simulink model "TV_2017old"  (R2016a)
settings: Solver=FixedStepAuto  StartTime=0.0  StopTime=inf  FixedStep=0.001  RelTol=1e-3
PreLoadFcn:
  | TV_2017_parameters
values from neighbouring files (symbols this model uses):
  battery_voltage = single(530)    [HIL_parameters.m]    (also in HIL_parameters_2018.m; TV_2017_parameters.m; TV_2017_parameters_VD.m)
  car_params = Simulink_Car_params    [HIL_parameters.m]    (also in HIL_parameters_2018.m; TV_2017_parameters.m; TV_2017_parameters_VD.m)
  i_Diff = 16    [HIL_parameters.m]    (also in HIL_parameters_2018.m; TV_2017_parameters.m)
  Kp = 1    [HIL_parameters.m]    (also in HIL_parameters_2018.m; TV_2017_parameters.m; TV_2017_parameters_VD.m)
  motor_data = struct    [HIL_parameters.m]    (also in HIL_parameters_2018.m; TV_2017_parameters.m)
  powerLimitControl = Simulink_el    [HIL_parameters.m]    (also in HIL_parameters_2018.m; TV_2017_parameters.m; TV_2017_parameters_VD.m)
  settings = Simulink_Settings    [HIL_parameters.m]    (also in HIL_parameters_2018.m; TV_2017_parameters.m; TV_2017_parameters_VD.m)
  SpdC_BCC = 0    [HIL_parameters.m]    (also in HIL_parameters_2018.m; TV_2017_parameters.m; TV_2017_parameters_VD.m)
  Speed_Neg_sat = -21    [HIL_parameters.m]    (also in HIL_parameters_2018.m; TV_2017_parameters.m; TV_2017_parameters_VD.m)
  Speed_Pos_sat = 21    [HIL_parameters.m]    (also in HIL_parameters_2018.m; TV_2017_parameters.m; TV_2017_parameters_VD.m)
  SteeringAngleFL = [-23.80 -22.65 -21.50 -20.34 -19.18 -18.03 -16.86 -15.70 -14.53 -13.35 -12.18 -10.99 -9.80 -8.61 -7.40 -6.19 -4.97 -3.75 -2.51 -1.26 0 1.27 2.56 3.85 5.17 6.50 7.84 9.21 10.59 12.00 13.42 14.88 16.36 17.87 19.41 20.99 22.61 24.26 25.97 27.73 29.54]    [CarSetupAnalysis2018.m]    (also in HIL_parameters_2018.m; TV_2017_parameters.m; TV_2017_parameters_VD.m = [-24.129 -22.950 -21.772 -20.593 -19.413 -18.232 -17.050 -15)
  SteeringAngleFR = [-29.54 -27.73 -25.97 -24.26 -22.61 -20.99 -19.41 -17.87 -16.36 -14.88 -13.42 -12.00 -10.59 -9.21 -7.84 -6.50 -5.17 -3.85 -2.56 -1.27 0 1.26 2.51 3.75 4.97 6.19 7.40 8.61 9.80 10.99 12.18 13.35 14.53 15.70 16.86 18.03 19.18 20.34 21.50 22.65 23.80]    [CarSetupAnalysis2018.m]    (also in HIL_parameters_2018.m; TV_2017_parameters.m; TV_2017_parameters_VD.m = [-29.3050 -27.5340 -25.8140 -24.1410 -22.5110 -20.9180 -19.3)
  SteeringWhAngle = [-105 -99.75 -94.5 -89.25 -84 -78.75 -73.5 -68.25 -63 -57.75 -52.5 -47.25 -42 -36.75 -31.5 -26.25 -21.0 -15.75 -10.5 -5.25 0.0 5.25 10.50 15.75 21.00 26.25 31.50 36.75 42.00 47.25 52.50 57.75  63.00 68.25 73.50 78.75 84.00 89.25 94.50 99.75 105.00]    [TV_2017_parameters_VD.m]
  Tn_n = 0    [HIL_parameters.m]    (also in HIL_parameters_2018.m; TV_2017_parameters.m; TV_2017_parameters_VD.m)
  tractionControl = Simulink_tc    [HIL_parameters.m]    (also in HIL_parameters_2018.m; IterativeTractionControlTuning.m; TV_2017_parameters.m; TV_2017_parameters_VD.m)
  yawRateControl = Simulink_yawRate    [HIL_parameters.m]    (also in HIL_parameters_2018.m; TV_2017_parameters.m; TV_2017_parameters_VD.m)
undefined symbols (not defined in the file or in its folder): DiscIntNeverNeededParam, magnitude, speedEstimation, TC_Decr_Gas, TC_Derivative, TC_Incr_Gas, TC_On, TC_Relay_Off, TC_Relay_On
libraries: CarMaker4SL x274, simulink_extras x45, simulink x37, dspfdesign x2
(part 7 of 14)

== system TV_2017old/CarMaker/IPG Vehicle3/PowerTrain/Electric Powertrain/AMK RL ==
  Motor_speed_ref_in_RPM : Inport
  Whl_speed_rad_per_sec : Inport  Port=2
  "Torque_limit_pos " : Inport  Port=3
  Torque_limit_neg : Inport  Port=4
  Convert to RPM : Gain  Gain=60/(2*pi)
  Delay : Delay  DelayLength=3  InitialCondition=0
  Gain2 : Gain  Gain=-1
  Gear ratio : Gain  Gain=car_params.GR
  Gear ratio2 : Gain  Gain=car_params.GR
  Maximum torque output based on motor RPM : Lookup_n-D  NumberOfTableDimensions=1  BreakpointsForDimension1=motor_data.MaxTorqueBreakpoints  BreakpointsForDimension1Min=[0]  BreakpointsForDimension1Max=[20000]  Table=motor_data.MaxTorqueValues  ExtrapMethod=Clip  UseLastTableValue=on  InternalRulePriority=Speed  OutMin=[0]  OutMax=[21]  RndMeth=Simplest  InputSameDT=on
  Saturation : simulink/Discontinuities/Saturation Dynamic  OutMin=[]  OutMax=[]  OutDataTypeStr=Inherit: Same as second input  OutDataType=fixdt(1, 16)  OutScaling=2^-10  DoSatur=off
  Saturation Dynamic1 : simulink/Discontinuities/Saturation Dynamic  OutMin=[]  OutMax=[]  OutDataTypeStr=Inherit: Same as second input  OutDataType=fixdt(1, 16)  OutScaling=2^-10  DoSatur=off
  Speed PI 1 : simulink/Continuous/PID Controller  Controller=PI  TimeDomain=Discrete-time  SampleTime=-1  IntegratorMethod=Forward Euler  FilterMethod=Forward Euler  Form=Parallel  UseFilter=on  ControllerParametersSource=internal  P=Kp  I=Tn_n  D=0  N=100  InitialConditionSource=internal  InitialConditionForIntegrator=0  InitialConditionForFilter=0  ExternalReset=none  LimitOutput=on  UpperSaturationLimit=Speed_Pos_sat  LowerSaturationLimit=Speed_Neg_sat  LinearizeAsGain=off  AntiWindupMode=back-calculation  Kb=SpdC_BCC  TrackingMode=off  Kt=1  PParamMin=[]  PParamMax=[]  IParamMin=[]  IParamMax=[]  DParamMin=[]  DParamMax=[]  NParamMin=[]  NParamMax=[]  KbParamMin=[]  KbParamMax=[]  KtParamMin=[]  KtParamMax=[]  POutMin=[]  POutMax=[]  IOutMin=[]  IOutMax=[]  DOutMin=[]  DOutMax=[]  NOutMin=[]  NOutMax=[]  KbOutMin=[]  KbOutMax=[]  KtOutMin=[]  KtOutMax=[]  IntegratorOutMin=[]  IntegratorOutMax=[]  FilterOutMin=[]  FilterOutMax=[]  SumOutMin=[]  SumOutMax=[]  SumI1OutMin=[]  SumI1OutMax=[]  SumI2OutMin=[]  SumI2OutMax=[]  SumI3OutMin=[]  SumI3OutMax=[]  SumDOutMin=[]  SumDOutMax=[]  SaturationOutMin=[]  SaturationOutMax=[]  IntegratorContinuousStateAttributes=''  IntegratorStateMustResolveToSignalObject=off  IntegratorRTWStateStorageClass=Auto  FilterContinuousStateAttributes=''  FilterStateMustResolveToSignalObject=off  FilterRTWStateStorageClass=Auto  DifferentiatorICPrevScaledInput=0  DifferentiatorOutMin=[]  DifferentiatorOutMax=[]
  Sum : Sum  Inputs=|+-
  "Torque_Output " : Outport
  wires:
  Delay/1 -> "Torque_Output "/1
  Speed PI 1/1 -> Saturation/2
  Maximum torque output based on motor RPM/1 -> Saturation Dynamic1/1, Gain2/1
  Saturation Dynamic1/1 -> Gear ratio2/1
  Whl_speed_rad_per_sec/1 -> Gear ratio/1
  Gain2/1 -> Saturation Dynamic1/3
  Gear ratio2/1 -> Delay/1
  "Torque_limit_pos "/1 -> Saturation/1
  Torque_limit_neg/1 -> Saturation/3
  Motor_speed_ref_in_RPM/1 -> Sum/1
  Saturation/1 -> Saturation Dynamic1/2
  Sum/1 -> Speed PI 1/1
  Convert to RPM/1 -> Sum/2, Maximum torque output based on motor RPM/1
  Gear ratio/1 -> Convert to RPM/1

== system TV_2017old/CarMaker/IPG Vehicle3/PowerTrain/Electric Powertrain/AMK RR ==
  Motor_speed_ref_in_RPM : Inport
  Whl_speed_rad_per_sec : Inport  Port=2
  "Torque_limit_pos " : Inport  Port=3
  Torque_limit_neg : Inport  Port=4
  Convert to RPM : Gain  Gain=60/(2*pi)
  Delay : Delay  DelayLength=3  InitialCondition=0
  Gain2 : Gain  Gain=-1
  Gear ratio : Gain  Gain=car_params.GR
  Gear ratio2 : Gain  Gain=car_params.GR
  Maximum torque output based on motor RPM : Lookup_n-D  NumberOfTableDimensions=1  BreakpointsForDimension1=motor_data.MaxTorqueBreakpoints  BreakpointsForDimension1Min=[0]  BreakpointsForDimension1Max=[20000]  Table=motor_data.MaxTorqueValues  ExtrapMethod=Clip  UseLastTableValue=on  InternalRulePriority=Speed  OutMin=[0]  OutMax=[21]  RndMeth=Simplest  InputSameDT=on
  Saturation : simulink/Discontinuities/Saturation Dynamic  OutMin=[]  OutMax=[]  OutDataTypeStr=Inherit: Same as second input  OutDataType=fixdt(1, 16)  OutScaling=2^-10  DoSatur=off
  Saturation Dynamic1 : simulink/Discontinuities/Saturation Dynamic  OutMin=[]  OutMax=[]  OutDataTypeStr=Inherit: Same as second input  OutDataType=fixdt(1, 16)  OutScaling=2^-10  DoSatur=off
  Speed PI 1 : simulink/Continuous/PID Controller  Controller=PI  TimeDomain=Discrete-time  SampleTime=-1  IntegratorMethod=Forward Euler  FilterMethod=Forward Euler  Form=Parallel  UseFilter=on  ControllerParametersSource=internal  P=Kp  I=Tn_n  D=0  N=100  InitialConditionSource=internal  InitialConditionForIntegrator=0  InitialConditionForFilter=0  ExternalReset=none  LimitOutput=on  UpperSaturationLimit=Speed_Pos_sat  LowerSaturationLimit=Speed_Neg_sat  LinearizeAsGain=off  AntiWindupMode=back-calculation  Kb=SpdC_BCC  TrackingMode=off  Kt=1  PParamMin=[]  PParamMax=[]  IParamMin=[]  IParamMax=[]  DParamMin=[]  DParamMax=[]  NParamMin=[]  NParamMax=[]  KbParamMin=[]  KbParamMax=[]  KtParamMin=[]  KtParamMax=[]  POutMin=[]  POutMax=[]  IOutMin=[]  IOutMax=[]  DOutMin=[]  DOutMax=[]  NOutMin=[]  NOutMax=[]  KbOutMin=[]  KbOutMax=[]  KtOutMin=[]  KtOutMax=[]  IntegratorOutMin=[]  IntegratorOutMax=[]  FilterOutMin=[]  FilterOutMax=[]  SumOutMin=[]  SumOutMax=[]  SumI1OutMin=[]  SumI1OutMax=[]  SumI2OutMin=[]  SumI2OutMax=[]  SumI3OutMin=[]  SumI3OutMax=[]  SumDOutMin=[]  SumDOutMax=[]  SaturationOutMin=[]  SaturationOutMax=[]  IntegratorContinuousStateAttributes=''  IntegratorStateMustResolveToSignalObject=off  IntegratorRTWStateStorageClass=Auto  FilterContinuousStateAttributes=''  FilterStateMustResolveToSignalObject=off  FilterRTWStateStorageClass=Auto  DifferentiatorICPrevScaledInput=0  DifferentiatorOutMin=[]  DifferentiatorOutMax=[]
  Sum : Sum  Inputs=|+-
  "Torque_Output " : Outport
  wires:
  Gear ratio/1 -> Convert to RPM/1
  Convert to RPM/1 -> Maximum torque output based on motor RPM/1, Sum/2
  Sum/1 -> Speed PI 1/1
  Saturation/1 -> Saturation Dynamic1/2
  Motor_speed_ref_in_RPM/1 -> Sum/1
  Torque_limit_neg/1 -> Saturation/3
  "Torque_limit_pos "/1 -> Saturation/1
  Gear ratio2/1 -> Delay/1
  Gain2/1 -> Saturation Dynamic1/3
  Whl_speed_rad_per_sec/1 -> Gear ratio/1
  Saturation Dynamic1/1 -> Gear ratio2/1
  Maximum torque output based on motor RPM/1 -> Gain2/1, Saturation Dynamic1/1
  Speed PI 1/1 -> Saturation/2
  Delay/1 -> "Torque_Output "/1

== system TV_2017old/CarMaker/IPG Vehicle3/PowerTrain/Electric Powertrain/E-Gas // E-Motor ==
  VC.Gas : Inport
  Constant : Constant  Value=TC_On
  Constant1 : Constant  Value=TC_On
  E-Motor Mapping RL : Lookup2D  RowIndex=FSE_M85(1,2:end)  ColumnIndex=FSE_M85(2:end,1)  Table=FSE_M85(2:end,2:end)'  LookUpMeth=Interpolation-Use End Values
  E-Motor Mapping RR : Lookup2D  RowIndex=FSE_M85(1,2:end)  ColumnIndex=FSE_M85(2:end,1)  Table=FSE_M85(2:end,2:end)'  LookUpMeth=Interpolation-Use End Values
  Electronic Gas Pedal RL : Subsystem
  Electronic Gas Pedal RR : Subsystem
  Gain : Gain
  Gain1 : Gain
  Rotation RL : Subsystem
  Rotation RR : Subsystem
  Transfer Fcn : TransferFcn  Denominator=[0.015 1]
  Transfer Fcn1 : TransferFcn  Denominator=[0.015 1]
  Trq_RL : Outport
  Trq_RR : Outport  Port=2
  wires:
  Rotation RL/1(Engine_rot_RL) -> E-Motor Mapping RL/1
  Constant/1 -> Electronic Gas Pedal RL/1(TC_On)
  Electronic Gas Pedal RL/1(Motor_Gas_RL) -> E-Motor Mapping RL/2
  VC.Gas/1 -> Electronic Gas Pedal RL/2(VC.Gas), Electronic Gas Pedal RR/2(VC.Gas)
  Constant1/1 -> Electronic Gas Pedal RR/1(TC_On)
  E-Motor Mapping RL/1 -> Transfer Fcn/1
  Transfer Fcn/1 -> Gain/1
  Gain/1 -> Trq_RL/1
  Rotation RR/1(Engine_rot_RR) -> E-Motor Mapping RR/1
  Electronic Gas Pedal RR/1(Motor_Gas_RR) -> E-Motor Mapping RR/2
  Transfer Fcn1/1 -> Gain1/1
  E-Motor Mapping RR/1 -> Transfer Fcn1/1
  Gain1/1 -> Trq_RR/1

== system TV_2017old/CarMaker/IPG Vehicle3/PowerTrain/Electric Powertrain/Gas Pedal ==
  Clock : Clock
  Constant : Constant  Value=0
  Constant1 : Constant
  Fcn : Fcn  Expr=u==0
  Read CM Dict : CarMaker4SL/Read CM Dict  xname=Vhcl.Ignition  xsync=off
  Read CM Dict2 : CarMaker4SL/Read CM Dict  xname=VC.Gas  xsync=off
  Switch : Switch
  Switch1 : Switch
  Write CM Dict : CarMaker4SL/Write CM Dict  xname=Vhcl.Ignition  xsync=off
  VC.Gas : Outport
  wires:
  Read CM Dict2/1 -> Switch/1
  Switch/1 -> VC.Gas/1
  Constant/1 -> Switch/3
  Switch1/1 -> Switch/2, Write CM Dict/1
  Read CM Dict/1 -> Switch1/3
  Constant1/1 -> Switch1/1
  Fcn/1 -> Switch1/2
  Clock/1 -> Fcn/1

== system TV_2017old/CarMaker/IPG Vehicle3/CarAndTrailer/Forces/Tires/TireFL ==
  note: Insert your tire model here.
  Sync_In : Inport
  Load : Inport  Port=2
  vxtrans : Inport  Port=3
  vytrans : Inport  Port=4
  Rim_rotv : Inport  Port=5
  Rim_turnv : Inport  Port=6
  InclinAngle : Inport  Port=7
  muRoad : Inport  Port=8
  Ground{1..11} (11 alike) : Ground
  Terminator{,1..6,12} (8 alike) : Terminator
  Slp : Outport
  Alpha : Outport  Port=2
  TurnSlp : Outport  Port=3
  rBelt_eff : Outport  Port=4
  vBelt : Outport  Port=5
  LongFrc : Outport  Port=6
  SideFrc : Outport  Port=7
  LoadFrc : Outport  Port=8
  OverturnTrq : Outport  Port=9
  RollResist : Outport  Port=10
  AlignTrq : Outport  Port=11
  wires:
  Ground11/1 -> vBelt/1
  Ground10/1 -> rBelt_eff/1
  Ground9/1 -> TurnSlp/1
  Rim_turnv/1 -> Terminator6/1
  Sync_In/1 -> Terminator12/1
  Ground2/1 -> Alpha/1
  Ground3/1 -> LongFrc/1
  Ground4/1 -> SideFrc/1
  Ground5/1 -> OverturnTrq/1
  vxtrans/1 -> Terminator1/1
  vytrans/1 -> Terminator2/1
  Rim_rotv/1 -> Terminator3/1
  InclinAngle/1 -> Terminator4/1
  muRoad/1 -> Terminator5/1
  Load/1 -> Terminator/1
  Ground1/1 -> Slp/1
  Ground6/1 -> LoadFrc/1
  Ground7/1 -> RollResist/1
  Ground8/1 -> AlignTrq/1

== system TV_2017old/CarMaker/IPG Vehicle3/CarAndTrailer/Forces/Tires/TireFR ==
  note: Insert your tire model here.
  Sync_In : Inport
  Load : Inport  Port=2
  vxtrans : Inport  Port=3
  vytrans : Inport  Port=4
  Rim_rotv : Inport  Port=5
  Rim_turnv : Inport  Port=6
  InclinAngle : Inport  Port=7
  muRoad : Inport  Port=8
  Ground{1..11} (11 alike) : Ground
  Terminator{,1..6,12} (8 alike) : Terminator
  Slp : Outport
  Alpha : Outport  Port=2
  TurnSlp : Outport  Port=3
  rBelt_eff : Outport  Port=4
  vBelt : Outport  Port=5
  LongFrc : Outport  Port=6
  SideFrc : Outport  Port=7
  LoadFrc : Outport  Port=8
  OverturnTrq : Outport  Port=9
  RollResist : Outport  Port=10
  AlignTrq : Outport  Port=11
  wires:
  Ground11/1 -> vBelt/1
  Ground10/1 -> rBelt_eff/1
  Ground9/1 -> TurnSlp/1
  Rim_turnv/1 -> Terminator6/1
  Sync_In/1 -> Terminator12/1
  Ground2/1 -> Alpha/1
  Ground3/1 -> LongFrc/1
  Ground4/1 -> SideFrc/1
  Ground5/1 -> OverturnTrq/1
  vxtrans/1 -> Terminator1/1
  vytrans/1 -> Terminator2/1
  Rim_rotv/1 -> Terminator3/1
  InclinAngle/1 -> Terminator4/1
  muRoad/1 -> Terminator5/1
  Load/1 -> Terminator/1
  Ground1/1 -> Slp/1
  Ground6/1 -> LoadFrc/1
  Ground7/1 -> RollResist/1
  Ground8/1 -> AlignTrq/1

== system TV_2017old/CarMaker/IPG Vehicle3/CarAndTrailer/Forces/Tires/TireRL ==
  note: Insert your tire model here.
  Sync_In : Inport
  Load : Inport  Port=2
  vxtrans : Inport  Port=3
  vytrans : Inport  Port=4
  Rim_rotv : Inport  Port=5
  Rim_turnv : Inport  Port=6
  InclinAngle : Inport  Port=7
  muRoad : Inport  Port=8
  Ground{1..11} (11 alike) : Ground
  Terminator{,1..6,12} (8 alike) : Terminator
  Slp : Outport
  Alpha : Outport  Port=2
  TurnSlp : Outport  Port=3
  rBelt_eff : Outport  Port=4
  vBelt : Outport  Port=5
  LongFrc : Outport  Port=6
  SideFrc : Outport  Port=7
  LoadFrc : Outport  Port=8
  OverturnTrq : Outport  Port=9
  RollResist : Outport  Port=10
  AlignTrq : Outport  Port=11
  wires:
  Ground11/1 -> vBelt/1
  Ground10/1 -> rBelt_eff/1
  Ground9/1 -> TurnSlp/1
  Rim_turnv/1 -> Terminator6/1
  Sync_In/1 -> Terminator12/1
  Ground2/1 -> Alpha/1
  Ground3/1 -> LongFrc/1
  Ground4/1 -> SideFrc/1
  Ground5/1 -> OverturnTrq/1
  vxtrans/1 -> Terminator1/1
  vytrans/1 -> Terminator2/1
  Rim_rotv/1 -> Terminator3/1
  InclinAngle/1 -> Terminator4/1
  muRoad/1 -> Terminator5/1
  Load/1 -> Terminator/1
  Ground1/1 -> Slp/1
  Ground6/1 -> LoadFrc/1
  Ground7/1 -> RollResist/1
  Ground8/1 -> AlignTrq/1

== system TV_2017old/CarMaker/IPG Vehicle3/CarAndTrailer/Forces/Tires/TireRR ==
  note: Insert your tire model here.
  Sync_In : Inport
  Load : Inport  Port=2
  vxtrans : Inport  Port=3
  vytrans : Inport  Port=4
  Rim_rotv : Inport  Port=5
  Rim_turnv : Inport  Port=6
  InclinAngle : Inport  Port=7
  muRoad : Inport  Port=8
  Ground{1..11} (11 alike) : Ground
  Terminator{,1..6,12} (8 alike) : Terminator
  Slp : Outport
  Alpha : Outport  Port=2
  TurnSlp : Outport  Port=3
  rBelt_eff : Outport  Port=4
  vBelt : Outport  Port=5
  LongFrc : Outport  Port=6
  SideFrc : Outport  Port=7
  LoadFrc : Outport  Port=8
  OverturnTrq : Outport  Port=9
  RollResist : Outport  Port=10
  AlignTrq : Outport  Port=11
  wires:
  Ground11/1 -> vBelt/1
  Ground10/1 -> rBelt_eff/1
  Ground9/1 -> TurnSlp/1
  Rim_turnv/1 -> Terminator6/1
  Sync_In/1 -> Terminator12/1
  Ground2/1 -> Alpha/1
  Ground3/1 -> LongFrc/1
  Ground4/1 -> SideFrc/1
  Ground5/1 -> OverturnTrq/1
  vxtrans/1 -> Terminator1/1
  vytrans/1 -> Terminator2/1
  Rim_rotv/1 -> Terminator3/1
  InclinAngle/1 -> Terminator4/1
  muRoad/1 -> Terminator5/1
  Load/1 -> Terminator/1
  Ground1/1 -> Slp/1
  Ground6/1 -> LoadFrc/1
  Ground7/1 -> RollResist/1
  Ground8/1 -> AlignTrq/1

== system TV_2017old/CarMaker/IPG Vehicle3/PowerTrain/Electric Powertrain/E-Gas // E-Motor/Electronic Gas Pedal RL ==
  TC_On : Inport
  VC.Gas : Inport  Port=2
  Define CM Dict : CarMaker4SL/Define CM Dict  xname=E_Gas_RL  xmono=off  xtype=Double4  xdvaplace=None  xnstates=0  xfirststate=0  xinitial=0
  Read CM Dict1 : CarMaker4SL/Read CM Dict  xname=E_Gas_RL  xsync=off
  Read CM Dict2 : CarMaker4SL/Read CM Dict  xname=Car.LongSlipRL  xsync=off
  Subsystem1 : Subsystem
  Switch : Switch
  Write CM Dict : CarMaker4SL/Write CM Dict  xname=E_Gas_RL  xsync=off
  Motor_Gas_RL : Outport
  wires:
  VC.Gas/1 -> Switch/3, Subsystem1/1(VC.Gas)
  Switch/1 -> Motor_Gas_RL/1
  TC_On/1 -> Switch/2
  Subsystem1/1(E_Gas) -> Write CM Dict/1, Switch/1
  Read CM Dict1/1 -> Subsystem1/2(E_Gas.)
  Read CM Dict2/1 -> Subsystem1/3(Car.LongSlip)

== system TV_2017old/CarMaker/IPG Vehicle3/PowerTrain/Electric Powertrain/E-Gas // E-Motor/Electronic Gas Pedal RR ==
  TC_On : Inport
  VC.Gas : Inport  Port=2
  Define CM Dict : CarMaker4SL/Define CM Dict  xname=E_Gas_RR  xmono=off  xtype=Double4  xdvaplace=None  xnstates=0  xfirststate=0  xinitial=0
  Read CM Dict1 : CarMaker4SL/Read CM Dict  xname=E_Gas_RR  xsync=off
  Read CM Dict2 : CarMaker4SL/Read CM Dict  xname=Car.LongSlipRR  xsync=off
  Subsystem1 : Subsystem
  Switch : Switch
  Write CM Dict : CarMaker4SL/Write CM Dict  xname=E_Gas_RR  xsync=off
  Motor_Gas_RR : Outport
  wires:
  TC_On/1 -> Switch/2
  Switch/1 -> Motor_Gas_RR/1
  VC.Gas/1 -> Switch/3, Subsystem1/1(VC.Gas)
  Subsystem1/1(E_Gas) -> Write CM Dict/1, Switch/1
  Read CM Dict2/1 -> Subsystem1/3(Car.LongSlip)
  Read CM Dict1/1 -> Subsystem1/2(E_Gas.)

== system TV_2017old/CarMaker/IPG Vehicle3/PowerTrain/Electric Powertrain/E-Gas // E-Motor/Rotation RL ==
  Gain : Gain  Gain=i_Diff
  Gain1 : Gain  Gain=60/(2*pi)
  Read CM Dict : CarMaker4SL/Read CM Dict  xname=Car.WheelSpd_RL  xsync=off
  Engine_rot_RL : Outport
  wires:
  Read CM Dict/1 -> Gain/1
  Gain/1 -> Gain1/1
  Gain1/1 -> Engine_rot_RL/1

== system TV_2017old/CarMaker/IPG Vehicle3/PowerTrain/Electric Powertrain/E-Gas // E-Motor/Rotation RR ==
  Gain : Gain  Gain=i_Diff
  Gain1 : Gain  Gain=60/(2*pi)
  Read CM Dict : CarMaker4SL/Read CM Dict  xname=Car.WheelSpd_RR  xsync=off
  Engine_rot_RR : Outport
  wires:
  Gain1/1 -> Engine_rot_RR/1
  Gain/1 -> Gain1/1
  Read CM Dict/1 -> Gain/1

== system TV_2017old/CarMaker/IPG Vehicle3/PowerTrain/Electric Powertrain/E-Gas // E-Motor/Electronic Gas Pedal RL/Subsystem1 ==
  VC.Gas : Inport
  E_Gas. : Inport  Port=2
  Car.LongSlip : Inport  Port=3
  Add : Sum
  Compare To Constant : simulink/Logic and Bit Operations/Compare To Constant  relop=>  const=TC_Derivative  OutDataTypeStr=uint8  ZeroCross=off
  Derivative : Derivative
  Fcn : Fcn  Expr=u >0.05
  Fcn1 : Fcn  Expr=u+TC_Incr_Gas
  Fcn2 : Fcn  Expr=u-TC_Decr_Gas
  Multiport Switch : MultiPortSwitch  DataPortOrder=Zero-based contiguous  zeroidx=on
  Relational Operator : RelationalOperator  Operator=<=
  Relay : Relay  OnSwitchValue=TC_Relay_On  OffSwitchValue=TC_Relay_Off
  S-R Flip-Flop : simulink_extras/Flip Flops/S-R Flip-Flop  initial_condition=0
  Saturation : Saturate  UpperLimit=1  LowerLimit=0
  Saturation1 : Saturate  UpperLimit=1  LowerLimit=0
  Switch : Switch  Criteria=u2 > Threshold
  Terminator : Terminator
  E_Gas : Outport
  wires:
  Car.LongSlip/1 -> Relay/1, Derivative/1, Fcn/1
  Relay/1 -> Add/1
  Derivative/1 -> Compare To Constant/1
  Compare To Constant/1 -> Add/2
  Add/1 -> Multiport Switch/1
  Multiport Switch/1 -> E_Gas/1
  VC.Gas/1 -> Relational Operator/1, [A]
  E_Gas./1 -> Relational Operator/2, Fcn1/1, Fcn2/1, Multiport Switch/3
  S-R Flip-Flop/2 -> Terminator/1
  S-R Flip-Flop/1 -> Switch/2
  Switch/1 -> Multiport Switch/2
  Fcn/1 -> S-R Flip-Flop/1
  Relational Operator/1 -> S-R Flip-Flop/2
  Fcn1/1 -> Saturation1/1
  Saturation1/1 -> Switch/1
  Fcn2/1 -> Saturation/1
  Saturation/1 -> Multiport Switch/4
  [A] -> Switch/3

== system TV_2017old/CarMaker/IPG Vehicle3/PowerTrain/Electric Powertrain/E-Gas // E-Motor/Electronic Gas Pedal RR/Subsystem1 ==
  VC.Gas : Inport
  E_Gas. : Inport  Port=2
  Car.LongSlip : Inport  Port=3
  Add : Sum
  Compare To Constant : simulink/Logic and Bit Operations/Compare To Constant  relop=>  const=TC_Derivative  OutDataTypeStr=uint8  ZeroCross=off
  Derivative : Derivative
  Fcn : Fcn  Expr=u >0.05
  Fcn1 : Fcn  Expr=u+TC_Incr_Gas
  Fcn2 : Fcn  Expr=u-TC_Decr_Gas
  Multiport Switch : MultiPortSwitch  DataPortOrder=Zero-based contiguous  zeroidx=on
  Relational Operator : RelationalOperator  Operator=<=  InputSameDT=on
  Relay : Relay  OnSwitchValue=TC_Relay_On  OffSwitchValue=TC_Relay_Off
  S-R Flip-Flop : simulink_extras/Flip Flops/S-R Flip-Flop  initial_condition=0
  Saturation : Saturate  UpperLimit=1  LowerLimit=0
  Saturation1 : Saturate  UpperLimit=1  LowerLimit=0
  Switch : Switch  Criteria=u2 > Threshold
  Terminator : Terminator
  E_Gas : Outport
  wires:
  Car.LongSlip/1 -> Relay/1, Derivative/1, Fcn/1
  Relay/1 -> Add/1
  Derivative/1 -> Compare To Constant/1
  Compare To Constant/1 -> Add/2
  Add/1 -> Multiport Switch/1
  Multiport Switch/1 -> E_Gas/1
  VC.Gas/1 -> Relational Operator/1, [A]
  E_Gas./1 -> Relational Operator/2, Fcn1/1, Fcn2/1, Multiport Switch/3
  S-R Flip-Flop/2 -> Terminator/1
  S-R Flip-Flop/1 -> Switch/2
  Switch/1 -> Multiport Switch/2
  Fcn/1 -> S-R Flip-Flop/1
  Relational Operator/1 -> S-R Flip-Flop/2
  Fcn1/1 -> Saturation1/1
  Saturation1/1 -> Switch/1
  Fcn2/1 -> Saturation/1
  Saturation/1 -> Multiport Switch/4
  [A] -> Switch/3

== matlab function TV_2017old/CarMaker/Control_System /Power Limit Torque Reduction Controller /Old powerlimiting /extractPower1 ==
  data: states input; power output; powerLimitControl parameter
function power = extractPower(states,powerLimitControl)
%#codegen


if (powerLimitControl.enable == uint32(1))
    power = states.power;
else
    power = single(0);
end

end

== matlab function TV_2017old/CarMaker/Control_System /Yaw Rate Controller /yawRateReference ==
  data: r_der_error output; r_error output; vx output; states input Bus: States; prev_r_error input; r_ref output; yawRateControl parameter; car_params parameter; r_lim output; ay_max output; settings parameter
function [r_der_error,r_error, vx, r_ref,r_lim,ay_max]...
          = yawrate_reference(states,prev_r_error, yawRateControl, car_params,settings)

%#codegen
updatefactor = single(1);
r_lim = single(0);
ay_max = single(0);
delta = states.wheel_angle;
delta_der = states.wheel_speed;
% If Ku is negative there will be a problem if the denominator approaches
% zero at high speeds
r_ref = (states.V_x/(yawRateControl.r_ref_tuning_param + yawRateControl.Ku*states.V_x^2))*tan(delta); %  tan

%r_ref = (states.V_x/(yawRateControl.r_ref_tuning_param*(1 + yawRateControl.Ku*states.V_x^2)))* delta;

%Fzi = [states.Fz_FL states.Fz_FR states.Fz_RL states.Fz_RR];
if yawRateControl.enable_r_ref_limit == 1
    r_lim = settings.mu*yawRateControl.mu_scaling_r_ref_limit*9.81/states.V_x;
    if abs(r_ref) > abs(r_lim)
        r_ref = r_lim*sign(r_ref);
    end
end

r = states.r;
r_error = prev_r_error*(1-updatefactor) + updatefactor*(r_ref-r);
r_ref_der = (states.ax*delta + states.V_x*delta_der)/yawRateControl.r_ref_tuning_param;
r_der_error = r_ref_der*yawRateControl.ref_weight - states.r_der*yawRateControl.meas_weight;

vx = states.V_x;
end

== matlab function TV_2017old/CarMaker/Control_System /Slip Rate Control /Traction Controllers/MATLAB Function1 ==
  data: states input Bus: States; SR_FL output; SR_FR output; SR_RL output; SR_RR output; T_req input; tractionControl parameter; Kp output; Ki output; settings parameter; T_tv input Bus: Ti_lim
function [SR_FL, SR_FR, SR_RL, SR_RR, Kp, Ki] = slipRatioAndGains(states, T_req, tractionControl, settings, T_tv)
%#codegen


SR_FL = states.SR_FL;
SR_FR = states.SR_FR;
SR_RL = states.SR_RL;
SR_RR = states.SR_RR;



if (states.V_x >= 0) 
    vx_kmh = states.V_x*3.6;
else
    vx_kmh = single(0);
end

    

a_kp = single((tractionControl.Kp_end - tractionControl.Kp_start) / tractionControl.lookup_speed_end_kmh);
a_ki = single((tractionControl.Ki_end - tractionControl.Ki_start) / tractionControl.lookup_speed_end_kmh);



if ( ( (T_req + 0.0001) > 0) && (vx_kmh < tractionControl.full_gain_limit_kmh) )   
    Kp = min( (a_kp*max(0,vx_kmh) + tractionControl.Kp_start), tractionControl.Kp_end)  * abs(T_req)/(settings.max_motor_torque*4);
    Ki = min( (a_ki*max(0,vx_kmh) + tractionControl.Ki_start), tractionControl.Ki_end)  * abs(T_req)/(settings.max_motor_torque*4);
else
    Kp = min( (a_kp*max(0,vx_kmh) + tractionControl.Kp_start), tractionControl.Kp_end);
    Ki = min( (a_ki*max(0,vx_kmh) + tractionControl.Ki_start), tractionControl.Ki_end);
end

end






% This one solves starting from 0 kmh with the driver controlling the
% throttle. This statement reduces the gains according to the requested
% torque, to avoid oscillating torque output


% if ( ( (T_req + 0.0001) > 0) && (vx_kmh < tractionControl.full_gain_limit_kmh) )   
%     Kp_driving = min( (a_kp*max(0,vx_kmh) + tractionControl.Kp_start), tractionControl.Kp_end)  * abs(T_req)/(settings.max_motor_torque*4);
%     Ki_driving = min( (a_ki*max(0,vx_kmh) + tractionControl.Ki_start), tractionControl.Ki_end)  * abs(T_req)/(settings.max_motor_torque*4);
%     Kp_FL = Kp_driving;
%     Kp_FR = Kp_driving;
%     Kp_RL = Kp_driving;
%     Kp_RR = Kp_driving;
%     
%     Ki_FL = Ki_driving;
%     Ki_FR = Ki_driving;
%     Ki_RL = Ki_driving;
%     Ki_RR = Ki_driving;
%     %Kp = min( (a_kp*max(0,vx_kmh) + tractionControl.Kp_start), tractionControl.Kp_end)  * abs(T_req)/(settings.max_motor_torque*4);
%     %Ki = min( (a_ki*max(0,vx_kmh) + tractionControl.Ki_start), tractionControl.Ki_end)  * abs(T_req)/(settings.max_motor_torque*4);
% 
% % T_req positive and speed over full gain limit
% elseif ( ( (T_req + 0.0001) > 0) && (vx_kmh > tractionControl.full_gain_limit_kmh))
%     Kp_driving = min( (a_kp*max(0,vx_kmh) + tractionControl.Kp_start), tractionControl.Kp_end);
%     Ki_driving = min( (a_ki*max(0,vx_kmh) + tractionControl.Ki_start), tractionControl.Ki_end);
%     Kp_FL = Kp_driving;
%     Kp_FR = Kp_driving;
%     Kp_RL = Kp_driving;
%     Kp_RR = Kp_driving;
%     
%     Ki_FL = Ki_driving;
%     Ki_FR = Ki_driving;
%     Ki_RL = Ki_driving;
%     Ki_RR = Ki_driving;    
% else   
%     Kp_FL = min( (a_kp*max(0,vx_kmh) + tractionControl.Kp_start), tractionControl.Kp_end);
%     Kp_FR = min( (a_kp*max(0,vx_kmh) + tractionControl.Kp_start), tractionControl.Kp_end);
%     Kp_RL = min( (a_kp*max(0,vx_kmh) + tractionControl.Kp_start), tractionControl.Kp_end);
%     Kp_RR = min( (a_kp*max(0,vx_kmh) + tractionControl.Kp_start), tractionControl.Kp_end);
%     
%     Ki_FL = min( (a_ki*max(0,vx_kmh) + tractionControl.Ki_start), tractionControl.Ki_end);
%     Ki_FR = min( (a_ki*max(0,vx_kmh) + tractionControl.Ki_start), tractionControl.Ki_end);
%     Ki_RL = min( (a_ki*max(0,vx_kmh) + tractionControl.Ki_start), tractionControl.Ki_end);
%     Ki_RR = min( (a_ki*max(0,vx_kmh) + tractionControl.Ki_start), tractionControl.Ki_end);
%     
%     %Kp = tractionControl.Kp_braking;
%     %Ki = tractionControl.Ki_braking;
% end
% 
% if ( (T_tv.FL < 0) || (T_tv.FR < 0) || (T_tv.RL < 0) || (T_tv.RR < 0) )
%     Kp = tractionControl.Kp_braking;
%     Ki = tractionControl.Ki_braking;
% end

== matlab function TV_2017old/CarMaker/Control_System /MATLAB Function3 ==
  data: Ti input Bus: Ti_lim; states input; Ti_pos output Bus: Ti_pos; Ti_neg output Bus: Ti_neg; wi_setpoints output Bus: wi_set; settings parameter; car_params parameter; overTorque output
function [Ti_pos, Ti_neg, wi_setpoints, overTorque] = setPointCalculation(Ti,states,settings,car_params)
%#codegen

%Conversion factor to calculate RPM limits based on speed limits
%v_to_motor_RPM = single(60*car_params.GR/(2*pi*car_params.r_eff));
overTorque = int8(0);
r = car_params.r_eff;
GR = car_params.GR;
scale_factor = 5;
not_in_use = settings.RPM_scaling;
max_rpm = settings.max_RPM;
KERS_RPM_setpoint = settings.KERS_motor_RPM_setpoint;
%scaled_RPM_lim_pos = states.V_x* (60/2*pi*r)*scale_factor;
v_x = states.V_x;
if v_x>5;
    scaled_RPM_lim_pos =  min([max_rpm ,GR*v_x* (60/2*pi*r)*scale_factor]);
else
   scaled_RPM_lim_pos = single( min([max_rpm ,GR*5* (60/2*pi*r)*scale_factor]));
end


if max([Ti.FL Ti.FR Ti.RL Ti.RR]) > (21+0.0001)
    %this is bad
    overTorque = int8(1);
end



 %***************** FL *********** 

if  (Ti.FL <= 0)  
    Ti_pos.FL = int16(0);
    Ti_neg.FL = int16(max(-settings.max_motor_brake_torque/car_params.Mn, Ti.FL/car_params.Mn));
    wi_setpoints.FL = int16(KERS_RPM_setpoint);

elseif Ti.FL > 0
    Ti_pos.FL = int16(min(21/car_params.Mn , Ti.FL/car_params.Mn));
    Ti_neg.FL = int16(0);
    wi_setpoints.FL = int16(max_rpm);  
else
    Ti_pos.FL = int16(0);
    Ti_neg.FL = int16(0);
    wi_setpoints.FL = int16(1); 
end

%***************** FR ************

if  (Ti.FR <= 0)
    Ti_pos.FR = int16(0);
    Ti_neg.FR = int16(max(-settings.max_motor_brake_torque/car_params.Mn, Ti.FR/car_params.Mn));
    wi_setpoints.FR = int16(KERS_RPM_setpoint);

elseif Ti.FR > 0        
    Ti_pos.FR = int16( min(21/car_params.Mn , Ti.FR/car_params.Mn));
    Ti_neg.FR = int16(0);
    wi_setpoints.FR = int16(max_rpm);  
else
    Ti_pos.FR = int16(0);
    Ti_neg.FR = int16(0);
    wi_setpoints.FR = int16(1); 
end
%***************** RL ************
if  (Ti.RL <= 0)
    Ti_pos.RL = int16(0);
    Ti_neg.RL = int16(max(-settings.max_motor_brake_torque/car_params.Mn, Ti.RL/car_params.Mn));
    wi_setpoints.RL = int16(KERS_RPM_setpoint);

elseif Ti.RL > 0
    Ti_pos.RL = int16(min(21/car_params.Mn , Ti.RL/car_params.Mn));
    Ti_neg.RL = int16(0);
    wi_setpoints.RL = int16(max_rpm);  
else
    Ti_pos.RL = int16(0);
    Ti_neg.RL = int16(0);
    wi_setpoints.RL = int16(1); 
end

%***************** RR ************
if (Ti.RR <= 0)
    Ti_pos.RR = int16(0);
    Ti_neg.RR = int16(max(-settings.max_motor_brake_torque/car_params.Mn, Ti.RR/car_params.Mn));
    wi_setpoints.RR = int16(KERS_RPM_setpoint);

elseif Ti.RR > 0
    Ti_pos.RR = int16(min(21/car_params.Mn , Ti.RR/car_params.Mn));
    Ti_neg.RR = int16(0);
    wi_setpoints.RR = int16(max_rpm);  
else
    Ti_pos.RR = int16(0);
    Ti_neg.RR = int16(0);
    wi_setpoints.RR = int16(1); 
end
end



% _________________________________________________________________________________________  
% 
% %***************** FL ************
% if dynamic_rpm ==1
%     if  (Ti.FL <= 0)  
%         Ti_pos.FL = int16(0);
%         Ti_neg.FL = int16(max(-settings.max_motor_brake_torque/car_params.Mn, Ti.FL/car_params.Mn));
%         wi_setpoints.FL = int16(KERS_RPM_setpoint);
% 
%     elseif Ti.FL > 0 
%         Ti_pos.FL = int16( Ti.FL/car_params.Mn);
%         Ti_neg.FL = int16(0);
%         wi_setpoints.FL = int16(scaled_RPM_lim_pos);  
%     else
%         Ti_pos.FL = int16(0);
%         Ti_neg.FL = int16(0);
%         wi_setpoints.FL = int16(2); 
%     end
% 
%     %***************** FR ************
% 
%     if  (Ti.FR <= 0)
%         Ti_pos.FR = int16(0);
%         Ti_neg.FR = int16(max(-settings.max_motor_brake_torque/car_params.Mn, Ti.FR/car_params.Mn));
%         wi_setpoints.FR = int16(KERS_RPM_setpoint);
% 
%     elseif Ti.FR > 0
%         Ti_pos.FR = int16( Ti.FR/car_params.Mn);
%         Ti_neg.FR = int16(0);
%         wi_setpoints.FR = int16(scaled_RPM_lim_pos);  
%     else
%         Ti_pos.FR = int16(0);
%         Ti_neg.FR = int16(0);
%         wi_setpoints.FR = int16(2); 
%     end
%     %***************** RL ************
%     if  (Ti.RL <= 0)
%         Ti_pos.RL = int16(0);
%         Ti_neg.RL = int16(max(-settings.max_motor_brake_torque/car_params.Mn, Ti.RL/car_params.Mn));
%         wi_setpoints.RL = int16(KERS_RPM_setpoint);
% 
%     elseif Ti.RL > 0
%         Ti_pos.RL = int16( Ti.RL/car_params.Mn);
%         Ti_neg.RL = int16(0);
%         wi_setpoints.RL = int16(scaled_RPM_lim_pos);  
%     else
%         Ti_pos.RL = int16(0);
%         Ti_neg.RL = int16(0);
%         wi_setpoints.RL = int16(2); 
%     end
% 
%     %***************** RR ************
%     if (Ti.RR <= 0)
%         Ti_pos.RR = int16(0);
%         Ti_neg.RR = int16(max(-settings.max_motor_brake_torque/car_params.Mn, Ti.RR/car_params.Mn));
%         wi_setpoints.RR = int16(KERS_RPM_setpoint);
% 
%     elseif Ti.RR > 0
%         Ti_pos.RR = int16( Ti.RR/car_params.Mn);
%         Ti_neg.RR = int16(0);
%         wi_setpoints.RR = int16(scaled_RPM_lim_pos);  
%     else
%         Ti_pos.RR = int16(0);
%         Ti_neg.RR = int16(0);
%         wi_setpoints.RR = int16(2); 
%     end
%     
%     
% else
%     
%     
    
  % _________________________________________________________________________________________  
% % The RPM at which KERS is turned off
% RPM_limit_low = settings.KERS_speed_limit_hyst_low*v_to_motor_RPM;
% 
% % The RPM at which KERS is allowed again
% RPM_limit_high = settings.KERS_speed_limit_hyst_high*v_to_motor_RPM;
% 
% 
%    persistent firstIteration;
%    persistent KERS_ALLOWED_FL;
%    persistent KERS_ALLOWED_FR;
%    persistent KERS_ALLOWED_RL;
%    persistent KERS_ALLOWED_RR;
%    
%    
%    % Hysteresis on regenerative input based on RPM to avoid oscillation around 
%    % allowed KERS RPM 
%    if isempty(firstIteration)
%       firstIteration = 2; % Avoid overflow in the register and count 1 again
%       KERS_ALLOWED_FL = uint32(0);
%       KERS_ALLOWED_FR = uint32(0);
%       KERS_ALLOWED_RL = uint32(0);
%       KERS_ALLOWED_RR = uint32(0);
%    else
%        
%        %Hysteris around the minimum RPM Set point
%        if     ( (KERS_ALLOWED_FL == 0) && (states.RPM_FL > RPM_limit_high) )
%            KERS_ALLOWED_FL = uint32(1);
%        elseif ( (KERS_ALLOWED_FL == 1) && (states.RPM_FL < RPM_limit_low) )
%            KERS_ALLOWED_FL = uint32(0);
%        end
%        if     ( (KERS_ALLOWED_FR == 0) && (states.RPM_FR > RPM_limit_high) )
%            KERS_ALLOWED_FR = uint32(1);
%        elseif ( (KERS_ALLOWED_FR == 1) && (states.RPM_FR < RPM_limit_low) )
%            KERS_ALLOWED_FR = uint32(0);
%        end
%        if     ( (KERS_ALLOWED_RL == 0) && (states.RPM_RL > RPM_limit_high) )
%            KERS_ALLOWED_RL = uint32(1);
%        elseif ( (KERS_ALLOWED_RL == 1) && (states.RPM_RL < RPM_limit_low) )
%            KERS_ALLOWED_RL = uint32(0);
%        end
%        if     ( (KERS_ALLOWED_RR == 0) && (states.RPM_RR > RPM_limit_high) )
%            KERS_ALLOWED_RR = uint32(1);
%        elseif ( (KERS_ALLOWED_RR == 1) && (states.RPM_RR < RPM_limit_low) )
%            KERS_ALLOWED_RR = uint32(0);
%        end
%        
%        % Hysteresis around maximum RPM ? 
%        
%    end   
%       
% %***************** FL ************
% 
% if ( (Ti.FL <= 0) && (KERS_ALLOWED_FL == 1) ) 
%     Ti_pos.FL = int16(0);
%     Ti_neg.FL = int16( Ti.FL/car_params.Mn);
%     wi_setpoints.FL = int16(KERS_RPM_setpoint);
% elseif ( (Ti.FL <= 0) && (KERS_ALLOWED_FL == 0) )
%     Ti_pos.FL = int16(0);
%     Ti_neg.FL = int16(0);
%     wi_setpoints.FL = int16(0);
% elseif Ti.FL > 0
%     Ti_pos.FL = int16( Ti.FL/car_params.Mn);
%     Ti_neg.FL = int16(0);
%     wi_setpoints.FL = int16(max_rpm);  
% else
%     Ti_pos.FL = int16(0);
%     Ti_neg.FL = int16(0);
%     wi_setpoints.FL = int16(0); 
% end
% 
% %***************** FR ************
% 
% if ( (Ti.FR <= 0) && (KERS_ALLOWED_FR == 1) ) 
%     Ti_pos.FR = int16(0);
%     Ti_neg.FR = int16( Ti.FR/car_params.Mn);
%     wi_setpoints.FR = int16(KERS_RPM_setpoint);
% elseif ( (Ti.FR <= 0) && (KERS_ALLOWED_FR == 0) )
%     Ti_pos.FR = int16(0);
%     Ti_neg.FR = int16(0);
%     wi_setpoints.FR = int16(0);
% elseif Ti.FR > 0
%     Ti_pos.FR = int16( Ti.FR/car_params.Mn);
%     Ti_neg.FR = int16(0);
%     wi_setpoints.FR = int16(max_rpm);  
% else
%     Ti_pos.FR = int16(0);
%     Ti_neg.FR = int16(0);
%     wi_setpoints.FR = int16(0); 
% end
% %***************** RL ************
% if ( (Ti.RL <= 0) && (KERS_ALLOWED_RL == 1) ) 
%     Ti_pos.RL = int16(0);
%     Ti_neg.RL = int16( Ti.RL/car_params.Mn);
%     wi_setpoints.RL = int16(KERS_RPM_setpoint);
% elseif ( (Ti.RL <= 0) && (KERS_ALLOWED_RL == 0) )
%     Ti_pos.RL = int16(0);
%     Ti_neg.RL = int16(0);
%     wi_setpoints.RL = int16(0);
% elseif Ti.RL > 0
%     Ti_pos.RL = int16( Ti.RL/car_params.Mn);
%     Ti_neg.RL = int16(0);
%     wi_setpoints.RL = int16(max_rpm);  
% else
%     Ti_pos.RL = int16(0);
%     Ti_neg.RL = int16(0);
%     wi_setpoints.RL = int16(0); 
% end
% 
% %***************** RR ************
% if ( (Ti.RR <= 0) && (KERS_ALLOWED_RR == 1) ) 
%     Ti_pos.RR = int16(0);
%     Ti_neg.RR = int16( Ti.RR/car_params.Mn);
%     wi_setpoints.RR = int16(KERS_RPM_setpoint);
% elseif ( (Ti.RR <= 0) && (KERS_ALLOWED_RR == 0) )
%     Ti_pos.RR = int16(0);
%     Ti_neg.RR = int16(0);
%     wi_setpoints.RR = int16(0);
% elseif Ti.RR > 0
%     Ti_pos.RR = int16( Ti.RR/car_params.Mn);
%     Ti_neg.RR = int16(0);
%     wi_setpoints.RR = int16(max_rpm);  
% else
%     Ti_pos.RR = int16(0);
%     Ti_neg.RR = int16(0);
%     wi_setpoints.RR = int16(0); 
% end
% 
% end

== matlab function TV_2017old/CarMaker/Control_System /Yaw Rate Controller /gainScheduling ==
  data: Kd output; vx_kmh input; Kp output; Ki output; yawRateControl parameter
function [Kd, Kp, Ki] = gainScheduling(vx_kmh,yawRateControl)
%#codegen
if (vx_kmh <= 0)
    vx_kmh = single(0);
end


% a_kp = single((yawRateControl.Kp_end - yawRateControl.Kp_start) / yawRateControl.lookup_speed_end_kmh);
% a_ki = single((yawRateControl.Ki_end - yawRateControl.Ki_start) / yawRateControl.lookup_speed_end_kmh);
% a_kd = single((yawRateControl.Kd_end - yawRateControl.Kd_start) / yawRateControl.lookup_speed_end_kmh);
% 
% if (vx_kmh <= 0)
%     vx_kmh = single(0);
% end
% 
% Kp = min( (a_kp*max(0.1,vx_kmh) + yawRateControl.Kp_start), yawRateControl.Kp_end);
% 
% Ki = min( (a_ki*max(0.1,vx_kmh) + yawRateControl.Ki_start), yawRateControl.Ki_end);
% 
% Kd = min( (a_kd*max(0.1,vx_kmh) + yawRateControl.Kd_start), yawRateControl.Kd_end);
% 
% end

Kp_values = [yawRateControl.Kp_start yawRateControl.Kp_start  yawRateControl.Kp_end yawRateControl.Kp_end];
Kp_speeds = [0 yawRateControl.lookup_speed_end_kmh (yawRateControl.lookup_speed_end_kmh+20)  115];

Ki_values = [yawRateControl.Ki_start yawRateControl.Ki_start  yawRateControl.Ki_end yawRateControl.Ki_end];
Ki_speeds = [0 yawRateControl.lookup_speed_end_kmh (yawRateControl.lookup_speed_end_kmh+20)  115];

Kd_values = [yawRateControl.Kd_start yawRateControl.Kd_start  yawRateControl.Kd_end yawRateControl.Kd_end];
Kd_speeds = [0 yawRateControl.lookup_speed_end_kmh (yawRateControl.lookup_speed_end_kmh+20)  115];


Kp = interp1(Kp_speeds,Kp_values,vx_kmh); 
Ki = interp1(Ki_speeds,Ki_values,vx_kmh);
Kd = interp1(Kd_speeds,Kd_values,vx_kmh);


if Kp>= 0
    Kp = Kp;
elseif Kp < 0 
    Kp = Kp;
else
    Kp = single(0);
end

if Ki>= 0
    Ki = Ki;
elseif Ki < 0 
    Ki = Ki;
else
    Ki = single(0);
end

if Kd>= 0
    Kd = Kd;
elseif Kd < 0 
    Kd = Kd;
else
    Kd = single(0);
end



breakpoint = 1;

== matlab function TV_2017old/CarMaker/Control_System /OutputTelemetri ==
  data: states input; OutputTelemetri_control output Bus: OutputTelemetri_Control; T_req input; r_ref input; Mz_ref_to_telemetry input
function OutputTelemetri_control = OutputTelemetri(states, T_req, r_ref, Mz_ref_to_telemetry)
%#codegen

OutputTelemetri_control.T_req   = T_req;
OutputTelemetri_control.Mz_ref  = Mz_ref_to_telemetry;
OutputTelemetri_control.r_ref   = r_ref;
end

== matlab function TV_2017old/CarMaker/Control_System /Torque allocation 2017/Inverter temperature limiter ==
  data: states input; maxMotorTorque output Bus: maxMotorTorque; settings parameter; car_params parameter
function maxMotorTorque = maxMotorTorque_InvTemp(states,settings, car_params)
%#codegen
inv_FL_temp =int16(20);
inv_FR_temp =20;
inv_RL_temp =20;
inv_RR_temp =20;


% The inverters limits output torque based on internal temperature
mmt                 =  single(settings.max_motor_torque);
upper_max_temp      =  single(car_params.AMK_inverter_upper_max_temp);
cutoff_temp         =  single(car_params.AMK_inverter_cutoff_temp);

torque = [mmt, mmt, single(0)]; %breakpoints for lookup function
temp = [single(0), upper_max_temp, cutoff_temp];

inv_FL_temp = single(states.AMK_inverter_temp_FL);
inv_FR_temp = single(states.AMK_inverter_temp_FR);
inv_RL_temp = single(states.AMK_inverter_temp_RL);
inv_RR_temp = single(states.AMK_inverter_temp_RR);

%  y = interp1(xdata,ydata,x)
maxMotorTorque.mmt_FL = interp1(  temp , torque,  inv_FL_temp  );
maxMotorTorque.mmt_FR = interp1(  temp , torque,  inv_FR_temp  );
maxMotorTorque.mmt_RL = interp1(  temp , torque,  inv_RL_temp  );
maxMotorTorque.mmt_RR = interp1(  temp , torque,  inv_RR_temp  );

== matlab function TV_2017old/CarMaker/ECU input Sensors /estimated "Measured Power" based on Torque, RPM and datasheet IRL this is measured/MATLAB Function ==
  data: RPM_FL_IN input; RPM_FR_IN input; RPM_RL_IN input; RPM_RR_IN input; Pm_FL output; T input; T_FL output; RPM_FL output; Pm_FR output; T_FR output; RPM_FR output; Pm_RL output; T_RL output; RPM_RL output; Pm_RR output; T_RR output; RPM_RR output
function [Pm_FL, T_FL, RPM_FL,Pm_FR, T_FR, RPM_FR,Pm_RL, T_RL,...
          RPM_RL,Pm_RR, T_RR, RPM_RR] = powerMeasurement(RPM_FL_IN, RPM_FR_IN,RPM_RL_IN,RPM_RR_IN, T)
%#codegen

%Conversion from RPM to rad/s
c = single(2*pi/60);

T_FL = T.FL;
T_FR = T.FR;
T_RL = T.RL;
T_RR = T.RR;

RPM_FL = RPM_FL_IN;
RPM_FR = RPM_FR_IN;
RPM_RL = RPM_RL_IN;
RPM_RR = RPM_RR_IN;


Pm_FL = RPM_FL*c*T.FL;
Pm_FR = RPM_FR*c*T.FR;
Pm_RL = RPM_RL*c*T.RL;
Pm_RR = RPM_RR*c*T.RR;

== matlab function TV_2017old/CarMaker/Control_System /Torque allocation 2016/MATLAB Function ==
  data: states input; maxMotorTorque output Bus: maxMotorTorque; settings parameter
function maxMotorTorque = findMaxMotorTorque(states,settings)
%#codegen

% DC Voltage                             / states
% Max allowable current draw in total    /settings
% Load distribution                      /states

Fzi = [max(1,states.Fz_FL) max(1,states.Fz_FR) max(1,states.Fz_RL) max(1,states.Fz_RR)]';

switch settings.TV_Method
    case 1 % No negative torque
        alfa_r =  (Fzi(3) + Fzi(4)) / (Fzi(1) + Fzi(2) + Fzi(3) + Fzi(4));
    case 2 % with negative torque
        alfa_r =  (Fzi(3) + Fzi(4)) / (Fzi(1) + Fzi(2) + Fzi(3) + Fzi(4));
    case 3 % static 25 %
        alfa_r = single(0.5);
    case 4 % with negative torque, no Fz
        alfa_r = single(0.5);
    otherwise
        alfa_r = single(0.5);
end

RPM_to_angular = single(2*pi/60);
omega_FL = states.RPM_FL*RPM_to_angular;
omega_FR = states.RPM_FR*RPM_to_angular;
omega_RL = states.RPM_RL*RPM_to_angular;
omega_RR = states.RPM_RR*RPM_to_angular;

mmt = settings.max_motor_torque;
available_power = states.DC_voltage*settings.max_battery_discharge;

max_torque_front = min(mmt, (available_power*(1-alfa_r))/ (2 * max( max(1,omega_FL), max(1,omega_FR))) );
max_torque_rear = min(mmt, (available_power*alfa_r)     / (2 * max( max(1,omega_RL), max(1,omega_RR))) );
                      
maxMotorTorque.mmt_FL = max_torque_front;
maxMotorTorque.mmt_FR = max_torque_front;
maxMotorTorque.mmt_RL = max_torque_rear;
maxMotorTorque.mmt_RR = max_torque_rear;
maxMotorTorque.kers_allowed = single(0);
